simulink model "Multi_drones_intro_compare"  (R2021a)
settings: Solver=ode4  StartTime=0.0  StopTime=50  FixedStep=0.005  RelTol=1e-3
(part 7 of 7)

== matlab function Multi_drones_intro_compare/Controller 3/Controller/Attitude controller/Sliding mode differentiator/sliding mode differentiator ==
  data: z input; z_dot output; x_d input
function z_dot = sliding_diff(z,x_d)

%% This is the observer function that estimates the unknown reference derivatives

dimension = 3;

alpha_1 = 8;
alpha_2 = 10;
alpha_3 = 10;
alpha_4 = 12;

beta_xd = 0.1;          %%----- Might need change

xi_1 = z(dimension*0+1:dimension*1);
xi_2 = z(dimension*1+1:dimension*2);
xi_3 = z(dimension*2+1:dimension*3);
xi_4 = z(dimension*3+1:dimension*4);

%% tunning
nu_1 = -alpha_1 * power(beta_xd,1/4) * power(abs(xi_1-x_d),3/4) .* sign(xi_1-x_d) + xi_2;
nu_2 = -alpha_2 * power(beta_xd,1/3) * power(abs(xi_2-nu_1),2/3) .* sign(xi_2-nu_1) +xi_3;
nu_3 = -alpha_3 * power(beta_xd,1/2) * power(abs(xi_3-nu_2),1/2) .* sign(xi_3-nu_2) +xi_4;
nu_4 = -alpha_4 * beta_xd .* sign(xi_4-nu_3);

z_dot = [nu_1;nu_2;nu_3;nu_4];


end

== matlab function Multi_drones_intro_compare/Controller 3/Controller/Attitude controller/State selection ==
  data: states_i input; x_i_a output; v_i_a output
function [x_i_a, v_i_a] = state_select(states_i)

%% This function is built to select the attitude information
% states_i = [x_i_p; x_i_a; v_i_p; v_i_a]
x_i_a = states_i(4:6);
v_i_a = states_i(10:12);

end

== matlab function Multi_drones_intro_compare/Controller 3/Controller/Nominal control calculation ==
  data: u_nom_p output; states_i input; u_i input; u_nom_a output
function [u_nom_p, u_nom_a] = nominal_control_cal(states_i, u_i)

%% Introduction:
% This function aims to calculate the nominal control input in different
% loop and feed them to the observers

%% System parameter
m = [0.88,0.90,0.91,0.90,0.89,0.92] + 1.2;             %%%%%%%%%% Change if necc
R = [0.29, 0.31, 0.30, 0.32, 0.34, 0.33] ;

J_x = [1.25,1.25,1.25,1.25,1.25,1.25];
J_y = [1.25,1.25,1.25,1.25,1.25,1.25];
J_z = [2.5,2.5,2.5,2.5,2.5,2.5];

upsilon = [5,5,5,5,5,5]/100;       %% Reverse moment coefficent

%% Parameter selection
%% Parameter selection
serial_num = 3;         %% -- Change the serial number here

m_i = m(serial_num);
R_i = R(serial_num);

J_i_x = J_x(serial_num);
J_i_y = J_y(serial_num);
J_i_z = J_z(serial_num);

upsilon_i = upsilon(serial_num);

%% System states
x_i_a = states_i(4:6);

phi = x_i_a(1);
theta = x_i_a(2);
psi = x_i_a(3);

%% Control gain matrix
% Position loop
g_x_1 = cos(phi) * sin(theta) * cos(psi) + sin(phi) * sin(psi);
g_x_2 = cos(phi) * sin(theta) * sin(psi) - sin(phi) * cos(psi);
g_x_3 = cos(phi) * cos(theta);
g_p = [g_x_1; g_x_2; g_x_3]/m_i;

% Attitude loop
g_a = [0, -R_i/J_i_x, 0, R_i/J_i_x;
       -R_i/J_i_y, 0, R_i/J_i_y, 0;
       -upsilon_i/J_i_z, upsilon_i/J_i_z, -upsilon_i/J_i_z, upsilon_i/J_i_z];

%% Nominal control input
u_nom_p = g_p * ([1,1,1,1] * u_i);

u_nom_a = g_a * u_i;


end

== matlab function Multi_drones_intro_compare/Controller 3/Controller/Position controller1/Error calculation ==
  data: s_i_p output; x_i_p input; delta_x_p output; v_i_p input; Phi_i input; x_i_p_d input; v_i_p_d input; delta_v_p output
function [s_i_p, delta_x_p, delta_v_p] = error_cal(x_i_p, v_i_p, Phi_i, x_i_p_d, v_i_p_d)

%% Description
% This function is built to calculate the tracking errors and the sliding variable

%% Error states calculation
delta_x_p = x_i_p - x_i_p_d;
delta_v_p = v_i_p - v_i_p_d;

%% Sliding variable calculation
lambda_p = 2;           %% You may want to change this

s_i_p = delta_v_p + lambda_p * (delta_x_p - Phi_i);

end

== matlab function Multi_drones_intro_compare/Controller 3/Controller/Position controller1/Position loop observer/Error calculation ==
  data: x_i_p input; x_tilde_p output; v_i_p input; x_hat_p input; v_hat_p input; v_tilde_p output
function [x_tilde_p, v_tilde_p] = error_cal(x_i_p, v_i_p, x_hat_p, v_hat_p)

%% Description
% This function calculates the tracking error for the observer states

x_tilde_p = x_i_p - x_hat_p;
v_tilde_p = v_i_p - v_hat_p;

end

== matlab function Multi_drones_intro_compare/Controller 3/Controller/Position controller1/Position loop observer/MATLAB Function ==
  data: t input; w_hat_p output; w_hat_p input
function w_hat_p = smooth_intro(t, w_hat_p)

% if t<=2
%     w_hat_p = zeros(3,1);
% elseif (t>2 && t<=4)
%     w_hat_p = 0.25 * (t-2)^2 * w_hat_p;
% end

eta_2 = 4;
eta_3 = 2;

f = 1 - (exp(-eta_2 * (t - eta_3))/(1 + exp(-eta_2 * (t - eta_3))) );

w_hat_p = f * w_hat_p;

end

== matlab function Multi_drones_intro_compare/Controller 3/Controller/Position controller1/Position loop observer/Observation ==
  data: x_tilde_p input; u_hat_p output; v_tilde_p input; w_hat_p input; s_tilde_p input
function u_hat_p = observation(x_tilde_p, v_tilde_p, w_hat_p, s_tilde_p)

%% Description
% This function calculates the observation for position loop

%% Controller parameters
lambda_tilde = 2;           %% You may want to change that 
k_tilde = 4;
c_tilde = 4;

%% Final observation
u_hat_p = w_hat_p + lambda_tilde * v_tilde_p + c_tilde * s_tilde_p + k_tilde * x_tilde_p;

end

== matlab function Multi_drones_intro_compare/Controller 3/Controller/Position controller1/Position loop observer/Single Layer Neural network/Neural network output ==
  data: phi_net input; w_i output; W input
function w_i = neural_output(phi_net, W)

w_i = W' * phi_net;

end

== matlab function Multi_drones_intro_compare/Controller 3/Controller/Position controller1/Position loop observer/Single Layer Neural network/Update of neural weight ==
  data: phi_net input; W_dot output; esti_s input; W input
function W_dot = weight_update(phi_net, esti_s, W)

%% This function stands for the neural weight update procedure
eta_1 = 20;
eta_2 = 0.5;

W_dot = eta_1 * phi_net * esti_s' - eta_2 * norm(esti_s) * W;

% W_dot = eta_1 * phi_net * esti_s' - eta_2 * W;

% W_dot = eta_1 * phi_net * esti_s';


end

== matlab function Multi_drones_intro_compare/Controller 1/Controller/Attitude controller/Sliding mode differentiator/MATLAB Function ==
  data: ang_d output; z input; ang_d_dot output; ang_d_ddot output
function [ang_d, ang_d_dot, ang_d_ddot] = divide_n_send(z)

%% This function is for dividing the reference estimation for later design

dimension = 3;

ang_d = z(dimension*0+1 : dimension*1);
ang_d_dot = z(dimension*1+1 : dimension*2);
ang_d_ddot = z(dimension*2+1 : dimension*3);

end

== matlab function Multi_drones_intro_compare/Controller 3/Controller/Position controller1/Position loop observer/Single Layer Neural network/Weight initialisation ==
  data: W_0 output
function W_0 = weight_initial()

dimension = 6;

W_0= zeros(dimension*2,dimension/2);

end

== matlab function Multi_drones_intro_compare/Controller 1/Controller/Attitude controller/Attitude loop observer/MATLAB Function ==
  data: x_tilde_a input; s_tilde_a output; v_tilde_a input
function s_tilde_a = sliding_variable(x_tilde_a, v_tilde_a)

lambda_tilde = 3;
s_tilde_a = v_tilde_a + lambda_tilde * x_tilde_a;

end

== matlab function Multi_drones_intro_compare/Controller 1/Controller/Attitude controller/Sliding mode differentiator/sliding mode differentiator ==
  data: z input; z_dot output; x_d input
function z_dot = sliding_diff(z,x_d)

%% This is the observer function that estimates the unknown reference derivatives

dimension = 3;

alpha_1 = 8;
alpha_2 = 10;
alpha_3 = 10;
alpha_4 = 12;

beta_xd = 0.1;          %%----- Might need change

xi_1 = z(dimension*0+1:dimension*1);
xi_2 = z(dimension*1+1:dimension*2);
xi_3 = z(dimension*2+1:dimension*3);
xi_4 = z(dimension*3+1:dimension*4);

%% tunning
nu_1 = -alpha_1 * power(beta_xd,1/4) * power(abs(xi_1-x_d),3/4) .* sign(xi_1-x_d) + xi_2;
nu_2 = -alpha_2 * power(beta_xd,1/3) * power(abs(xi_2-nu_1),2/3) .* sign(xi_2-nu_1) +xi_3;
nu_3 = -alpha_3 * power(beta_xd,1/2) * power(abs(xi_3-nu_2),1/2) .* sign(xi_3-nu_2) +xi_4;
nu_4 = -alpha_4 * beta_xd .* sign(xi_4-nu_3);

z_dot = [nu_1;nu_2;nu_3;nu_4];


end

== matlab function Multi_drones_intro_compare/Controller 3/Controller/Position controller1/Position loop observer/Sliding variable calculation ==
  data: x_tilde_p input; s_tilde_p output; v_tilde_p input
function s_tilde_p = sliding_variable(x_tilde_p, v_tilde_p)

%% Description
% This function calculates the observation sliding surface

lambda_tilde = 2;           %% You may need to change the value
s_tilde_p = v_tilde_p + lambda_tilde * x_tilde_p;

end

== matlab function Multi_drones_intro_compare/Controller 3/Controller/Position controller1/Position loop observer/Virtual system ==
  data: u_hat_p input; v_hat_dot_p output; u_nom_p input
function v_hat_dot_p = fcn(u_hat_p, u_nom_p)

%% Description
% This function updates the states in the observer

%% Gravity constant
g = 9.81;

%% State update
v_hat_dot_p = u_nom_p + u_hat_p - [0;0;g];

end

== matlab function Multi_drones_intro_compare/Controller 3/Controller/Position controller1/Reference selection (Low) ==
  data: ref_x_p input; x_i_p_d output; v_i_p_d output; a_i_p_d output
function [x_i_p_d, v_i_p_d, a_i_p_d] = ref_selection(ref_x_p)

%% Description
% This function is built to separate the reference states

%% Reference dividing
x_i_p_d = ref_x_p(1:3);
v_i_p_d = ref_x_p(4:6);
a_i_p_d = ref_x_p(7:9);

end

== matlab function Multi_drones_intro_compare/Controller 3/Controller/Position controller1/State selection ==
  data: states_i input; x_i_p output; v_i_p output
function [x_i_p, v_i_p] = state_select(states_i)

%% Description
% This is the state selection model for the self-feedback
% x_ip, v_ip, x_ia, v_ia  -> x_i, v_i
% x_ip_d, v_ip_d, a_ip_d  -> ref_x_p
% psi_i_d  -> psi_i_d (not changing)

%% System states feedback
x_i = states_i(1:6);
v_i = states_i(7:12);

x_i_p = x_i(1:3);
v_i_p = v_i(1:3);

end
